simulink model "F16ASYM_Controlled"  (R2015a)
settings: Solver=ode3  SolverMode=SingleTasking  StartTime=0.0  StopTime=inf  FixedStep=T_sim  RelTol=1e-3
InitFcn:
  | load('NN_c_weights_Last_stable.mat')
StopFcn:
  | Final_results
values from neighbouring files (symbols this model uses):
  a1 = fitresult.p1    [Stall_protection.m]
  alpha_map_eval = ones(size(M_eval))*NaN    [Auto_trim_aid.m]    (also in Autotrim_maps.mat = [nan nan 0.277598136245 0.119432432992 0.0579479097061 0.027)
  beta_map_eval = ones(size(M_eval))*NaN    [Auto_trim_aid.m]    (also in Autotrim_maps.mat = [nan nan -0.00151549403324 0.00117807579006 -0.0052086799721)
  C_L_0 = fitresult.p2    [Stall_protection.m]
  G_eval = NaN*ones(size(M_sq,2),size(H_sq,2))    [Stall_protection.m]
  H_sq = unique(sort(H_sq))    [Stall_protection.m]
  H_sq_autotrim = min( F_envelope.H_1g):2000:max(F_envelope.H_1g)    [Auto_trim_aid.m]    (also in Autotrim_maps.mat = [0 2000 4000 6000 8000 10000 12000 14000 16000 18000])
  K_b_q_extrap_ACC = K_b_q_extrap    [RUN_ME.m]
  K_b_q_extrap_AoA = K_b_q_extrap    [RUN_ME.m]
  M_sq = unique(sort(M_sq))    [Stall_protection.m]
  M_sq_autotrim = 0:0.1:max(F_envelope.M_1g)    [Auto_trim_aid.m]    (also in Autotrim_maps.mat = [0 0.1 0.2 0.3 0.4 0.5 0.6 0.7 0.8 0.9 1 1.1 ... (21 element)
  T_sim = 0.02    [RUN_ME.m]
  tau_q_extrap_ACC = tau_q_extrap    [RUN_ME.m]
  tau_q_extrap_AoA = tau_q_extrap    [RUN_ME.m]
  velocity = M_eval(I,J)*a    [Auto_trim_aid.m]
undefined symbols (not defined in the file or in its folder): ACCEL, B, Earth, fi_flag_Simulink, GYRO, H_sq_sche, k_B, K_b_ACC_extrap, K_b_AoA_extrap, latitude, longitude, m, m_B, M_sq_sche, Model_used_flag, rad, s, sigbuilder_block, Stall_curve, tau_ACC_extrap, tau_AoA_extrap, Theta_1_roll_last, Theta_2_roll_last, Theta_3_roll_last, trim_control, trim_state, trim_throttle, V_Comp_A_w_z_last, V_Comp_last, V_Comp_last_ONE, V_long_lastA_w_z, V_long_lastAoA, V_roll_last, V_roll_lastMOD, V_yaw_last, W_Comp_A_w_z_last, W_Comp_last, W_long_lastA_w_z, W_long_lastAoA, W_roll_last, W_roll_lastMOD, W_yaw_last, WGS84
libraries: Adaptive_FaultTolerantControl x57, dspsigops x37, F16_Actuator_Library x14, commnoisgen2 x13, simulink x11, simulink_extras x10, dsparch4 x6, aerolibatmos2 x6, aerolibtransform2 x6, aerolibfltsims x3, dspvision x3, dspsnks4 x3
(part 5 of 14)

== system F16ASYM_Controlled/Primary Controller/P con  + Crossed NN + AWU+Lim + hand-over+Scheduling/P controller + adaptive Crossed NN + AWU+Lim    in ACC  ==
  A_w_z des : Inport
  AoA des (rad) : Inport  Port=2
  p des (rad/s) : Inport  Port=3
  beta des (rad) : Inport  Port=4
  Anti-windup A_w_z : Inport  Port=5
  Anti-windup AoA : Inport  Port=6
  Anti-windup beta : Inport  Port=7
  All measures : Inport  Port=8
  Anti-windup signals : Inport  Port=9
  Active : Inport  Port=10
  Body Rates Controller : Subsystem
  Bus Creator : BusCreator  Inputs=3
  Bus Creator1 : BusCreator  Inputs=2
  Bus Creator2 : BusCreator
  Bus Creator3 : BusCreator  Inputs=2
  Bus Selector3 : BusSelector  OutputSignals=signal1.SS meas (rad)
  Complete crossed On-line (adaptive) multi-layer NN: A_w_z : Subsystem  VariantControl=NN on A_w_z
  Display{,1..3,5..6} (6 alike) : Display
  "Display4 " : Display
  Lat_dir Dyn Inversion: beta_dot->r_c : Subsystem
  Long Dyn Inversion: alpha_dot ->q : Subsystem
  Longitudinal controller in A_w_z : Subsystem  VariantControl=Controller of A_w_z
  Memory : Memory  X0=[0,0,0]
  Physical limitation : Subsystem
  Ref Model and P Controller : Adaptive_FaultTolerantControl/Ref Model and P Controller  tau=0.45  y_i=trim_state(9)  K_f=1  K_b=5
  Scope1 : Scope
      settings: TimeRange=10  YMin=-1  YMax=1  SaveName=ScopeData27
  "Sigmoid " : Subsystem  mask{a=0.15}
      mask prompts: a "Sigmoid a param"
      mask TypeOptions a: a/Value
      mask Display:
      | x=-25:0.1:25;
      | 
      | y=(2.0 ./ (1.0 + exp(-a.*x))-1) ;
      | y2=zeros(size(x));
      | 
      | plot(x,y,x,y2);
      | 
      | text(-12,0.5, ['a= ',num2str(a)])
  Sum : Sum  Inputs=-+|
  Sum1 : Sum  Inputs=+-|
  Terminator1 : Terminator
  Angular acc des : Outport
  wires:
  Active/1 -> Complete crossed On-line (adaptive) multi-layer NN: A_w_z/Enable
  Physical limitation/1(v limted) -> Angular acc des/1
  Anti-windup signals/1 -> Complete crossed On-line (adaptive) multi-layer NN: A_w_z/4(AWU)
  Ref Model and P Controller/1 -> Lat_dir Dyn Inversion: beta_dot->r_c/1(beta_dot_c), Display5/1
  Complete crossed On-line (adaptive) multi-layer NN: A_w_z/1(v_ad^) -> Sum/1, Display2/1, Scope1/1  "v_ad^"
  "Sigmoid "/1(Out) -> Memory/1
  Anti-windup beta/1 -> Terminator1/1
  Bus Creator3/1 -> Bus Creator/3  "beta_r_chanel"
  Bus Creator2/1 -> Bus Creator3/2  "beta_chanel vars"
  Body Rates Controller/3(r_chanel vars) -> Bus Creator3/1  "r_chanel vars"
  Ref Model and P Controller/5 -> Bus Creator2/4  "K_b_beta"
  Ref Model and P Controller/4 -> Sum1/2
  Sum1/1 -> Bus Creator2/3  "beta_err"
  Ref Model and P Controller/3 -> Bus Creator2/2, Sum1/1  "beta_sf"
  Ref Model and P Controller/2 -> Bus Creator2/1  "beta_sf_dot"
  Bus Creator1/1 -> Bus Creator/1  "Long chanel"
  Longitudinal controller in A_w_z/1(A_chanel vars) -> Bus Creator1/1  "A_chanel vars"
  Body Rates Controller/1(q_chanel vars) -> Bus Creator1/2  "q_chanel_vars"
  Body Rates Controller/2(p_chanel vars) -> Bus Creator/2  "p_chanel_vars"
  Memory/1 -> Complete crossed On-line (adaptive) multi-layer NN: A_w_z/1(v_ad^ prev)
  Bus Creator/1 -> Complete crossed On-line (adaptive) multi-layer NN: A_w_z/3(NN variables)
  Body Rates Controller/4(Angular acc des (rad/s^2)) -> Sum/2, Display3/1  "v_p+v_dot_ff"
  All measures/1 -> Longitudinal controller in A_w_z/5(All meas), Long Dyn Inversion: alpha_dot ->q/2(All_meas), Bus Selector3/1, Lat_dir Dyn Inversion: beta_dot->r_c/2(All_meas), Body Rates Controller/4(All_meas), Physical limitation/2(all meas), Complete crossed On-line (adaptive) multi-layer NN: A_w_z/2(All_meas)
  Sum/1 -> Physical limitation/1(v comm), "Sigmoid "/1(In), "Display4 "/1  "v"
  A_w_z des/1 -> Longitudinal controller in A_w_z/1(A_w_z des)
  Anti-windup A_w_z/1 -> Longitudinal controller in A_w_z/3(Anti-windup A_w_z)
  Anti-windup AoA/1 -> Longitudinal controller in A_w_z/4(Anti-windup AoA)
  AoA des (rad)/1 -> Longitudinal controller in A_w_z/2(AoA des (rad))
  Longitudinal controller in A_w_z/2(alpha_dot_c) -> Display/1, Long Dyn Inversion: alpha_dot ->q/1(alpha_dot_c)
  beta des (rad)/1 -> Ref Model and P Controller/1
  Long Dyn Inversion: alpha_dot ->q/1(q_c) -> Display1/1, Body Rates Controller/2(q_ref)
  p des (rad/s)/1 -> Body Rates Controller/1(p_ref)
  Bus Selector3/1 -> Ref Model and P Controller/2  "<SS meas (rad)>"
  Lat_dir Dyn Inversion: beta_dot->r_c/1(r_c) -> Body Rates Controller/3(r_ref), Display6/1

== system F16ASYM_Controlled/Primary Controller/P con  + Crossed NN + AWU+Lim + hand-over+Scheduling/P controller + adaptive Crossed NN + AWU+Lim   in AoA ==
  A_w_z des : Inport
  AoA des (rad) : Inport  Port=2
  p des (rad/s) : Inport  Port=3
  beta des (rad) : Inport  Port=4
  Anti-windup A_w_z : Inport  Port=5
  Anti-windup AoA : Inport  Port=6
  Anti-windup beta : Inport  Port=7
  All measures : Inport  Port=8
  Anti-windup signals : Inport  Port=9
  Active : Inport  Port=10
  Body Rates Controller : Subsystem
  Bus Creator : BusCreator  Inputs=3
  Bus Creator1 : BusCreator  Inputs=2
  Bus Creator2 : BusCreator
  Bus Creator3 : BusCreator  Inputs=2
  Bus Selector3 : BusSelector  OutputSignals=signal1.SS meas (rad)
  Complete crossed On-line (adaptive) multi-layer NN: AoA : Subsystem  VariantControl=NN on AoA
  Display{,1..3,5..6} (6 alike) : Display
  "Display4 " : Display
  Lat_dir Dyn Inversion: beta_dot->r_c : Subsystem
  Long Dyn Inversion: alpha_dot ->q : Subsystem
  Longitudinal controller in AoA1 : Subsystem  VariantControl=Controller of AoA
  Memory : Memory  X0=[0,0,0]
  Physical limitation : Subsystem
  Ref Model and P Controller : Adaptive_FaultTolerantControl/Ref Model and P Controller  tau=0.45  y_i=trim_state(9)  K_f=1  K_b=5
  Scope1 : Scope
      settings: YMin=-8000  YMax=9000  SaveName=ScopeData27
  "Sigmoid " : Subsystem  mask{a=0.15}
      mask prompts: a "Sigmoid a param"
      mask TypeOptions a: a/Value
      mask Display:
      | x=-25:0.1:25;
      | 
      | y=(2.0 ./ (1.0 + exp(-a.*x))-1) ;
      | y2=zeros(size(x));
      | 
      | plot(x,y,x,y2);
      | 
      | text(-12,0.5, ['a= ',num2str(a)])
  Sum : Sum  Inputs=-+|
  Sum1 : Sum  Inputs=+-|
  Terminator1 : Terminator
  Angular acc des : Outport
  wires:
  Active/1 -> Complete crossed On-line (adaptive) multi-layer NN: AoA/Enable
  Anti-windup signals/1 -> Complete crossed On-line (adaptive) multi-layer NN: AoA/4(AWU)
  Physical limitation/1(v limted) -> Angular acc des/1
  Ref Model and P Controller/1 -> Lat_dir Dyn Inversion: beta_dot->r_c/1(beta_dot_c), Display5/1
  Complete crossed On-line (adaptive) multi-layer NN: AoA/1(v_ad^) -> Sum/1, Display2/1, Scope1/1  "v_ad^"
  "Sigmoid "/1(Out) -> Memory/1
  Anti-windup beta/1 -> Terminator1/1
  Bus Creator3/1 -> Bus Creator/3  "beta_r_chanel"
  Bus Creator2/1 -> Bus Creator3/2  "beta_chanel vars"
  Body Rates Controller/3(r_chanel vars) -> Bus Creator3/1  "r_chanel vars"
  Ref Model and P Controller/5 -> Bus Creator2/4  "K_b_beta"
  Ref Model and P Controller/4 -> Sum1/2
  Sum1/1 -> Bus Creator2/3  "beta_err"
  Ref Model and P Controller/3 -> Bus Creator2/2, Sum1/1  "beta_sf"
  Ref Model and P Controller/2 -> Bus Creator2/1  "beta_sf_dot"
  Bus Creator1/1 -> Bus Creator/1  "Long chanel"
  Longitudinal controller in AoA1/1(alpha_chanel vars) -> Bus Creator1/1  "alpha_chanel vars"
  Body Rates Controller/1(q_chanel vars) -> Bus Creator1/2  "q_chanel_vars"
  Body Rates Controller/2(p_chanel vars) -> Bus Creator/2  "p_chanel_vars"
  Memory/1 -> Complete crossed On-line (adaptive) multi-layer NN: AoA/1(v_ad^ prev)
  Bus Creator/1 -> Complete crossed On-line (adaptive) multi-layer NN: AoA/3(NN variables)
  Body Rates Controller/4(Angular acc des (rad/s^2)) -> Sum/2, Display3/1  "v_p+v_dot_ff"
  All measures/1 -> Longitudinal controller in AoA1/5(All meas), Long Dyn Inversion: alpha_dot ->q/2(All_meas), Bus Selector3/1, Lat_dir Dyn Inversion: beta_dot->r_c/2(All_meas), Body Rates Controller/4(All_meas), Physical limitation/2(all meas), Complete crossed On-line (adaptive) multi-layer NN: AoA/2(All_meas)
  Sum/1 -> Physical limitation/1(v comm), "Sigmoid "/1(In), "Display4 "/1  "v"
  A_w_z des/1 -> Longitudinal controller in AoA1/1(A_w_z des)
  Anti-windup A_w_z/1 -> Longitudinal controller in AoA1/3(Anti-windup A_w_z)
  Anti-windup AoA/1 -> Longitudinal controller in AoA1/4(Anti-windup AoA)
  AoA des (rad)/1 -> Longitudinal controller in AoA1/2(AoA des (rad))
  Longitudinal controller in AoA1/2(alpha_dot_c) -> Display/1, Long Dyn Inversion: alpha_dot ->q/1(alpha_dot_c)
  beta des (rad)/1 -> Ref Model and P Controller/1
  Long Dyn Inversion: alpha_dot ->q/1(q_c) -> Display1/1, Body Rates Controller/2(q_ref)
  p des (rad/s)/1 -> Body Rates Controller/1(p_ref)
  Bus Selector3/1 -> Ref Model and P Controller/2  "<SS meas (rad)>"
  Lat_dir Dyn Inversion: beta_dot->r_c/1(r_c) -> Body Rates Controller/3(r_ref), Display6/1

== system F16ASYM_Controlled/Primary Controller/P con  + Crossed NN + AWU+Lim + hand-over+Scheduling/Transitions Smoother  ==
  note: When changing here the time, be careful and change also
      | the denominator of the gains of the inputs of the integrators
  From AoA : Inport
  Indicator : Inport  Port=2
  From  ACC : Inport  Port=3
  "ACC -> AoA" : Saturate  UpperLimit=1  LowerLimit=0
  Abs : Abs
  Abs1 : Abs
  Add : Sum  Inputs=+-  OutDataTypeStr=double
  Add1 : Sum  Inputs=+-
  Add2 : Sum  Inputs=-+
  Add3 : Sum  Inputs=-+
  Add4 : Sum  Inputs=+-
  Add6 : Sum  Inputs=+-
  Add7 : Sum  Commented=on  Inputs=+-
  "AoA -> ACC" : Saturate  UpperLimit=0  LowerLimit=-1
  Divide : Product  Inputs=**
  Divide1 : Product  Inputs=**
  Gain1 : Gain  Gain=-1/1
  Gain2 : Gain  Gain=-1/1
  Integrator Limited1 : Integrator  ExternalReset=level  InitialConditionSource=external  LimitOutput=on  UpperSaturationLimit=100  LowerSaturationLimit=-100
  Integrator Limited2 : Integrator  ExternalReset=level  InitialConditionSource=external  LimitOutput=on  UpperSaturationLimit=100  LowerSaturationLimit=-100
  Logical Operator : Logic  Operator=NOT  IconShape=distinctive  AllPortsSameDT=off  OutDataTypeStr=boolean
  Logical Operator1 : Logic  Operator=NOT  IconShape=distinctive  AllPortsSameDT=off  OutDataTypeStr=boolean
  Logical Operator2 : Logic  Operator=NOT  IconShape=distinctive  AllPortsSameDT=off  OutDataTypeStr=boolean
  Sample and Hold{1..4} (4 alike) : dspsigops/Sample and Hold  trig=Either edge  initCond=0  latchinput=off
  Scope3 : Scope
      settings: SaveName=ScopeData36
  Scope4 : Scope
      settings: YMin=-0.08  YMax=0.02  SaveName=ScopeData37
  Switch : Switch  Threshold=0.5  InputSameDT=on
  Timer signal : Subsystem  mask{time_delay=1}
      mask prompts: time_delay "Time to delay (s)"
  Unit Delay : UnitDelay  SampleTime=-1
  Ang accels comm : Outport
  wires:
  Logical Operator2/1 -> Divide1/1
  Divide1/1 -> Add6/2, Scope3/1
  Divide/1 -> Scope4/1, Add4/2
  Logical Operator1/1 -> Divide/1
  Gain2/1 -> Integrator Limited2/1
  Gain1/1 -> Integrator Limited1/1
  Sample and Hold4/1 -> Add7/2
  "ACC -> AoA"/1 -> Sample and Hold4/Trigger, Sample and Hold3/Trigger
  Integrator Limited2/1 -> Divide1/2
  Add6/1 -> Switch/1
  Switch/1 -> Ang accels comm/1
  Logical Operator/1 -> Logical Operator1/1, Integrator Limited1/2, Logical Operator2/1, Integrator Limited2/2
  Add4/1 -> Switch/3
  Integrator Limited1/1 -> Divide/2
  Sample and Hold2/1 -> Add3/1
  Add3/1 -> Gain1/1
  Sample and Hold1/1 -> Integrator Limited1/3
  Add2/1 -> Sample and Hold1/1
  Abs/1 -> Sample and Hold2/Trigger, Sample and Hold1/Trigger
  From AoA/1 -> Add1/1, Add6/1, Add7/1, Add2/1, Sample and Hold2/1
  Add1/1 -> Sample and Hold3/1
  "AoA -> ACC"/1 -> Abs/1
  Add/1 -> Abs1/1, "ACC -> AoA"/1, "AoA -> ACC"/1
  From  ACC/1 -> Add1/2, Sample and Hold4/1, Add4/1, Add2/2, Add3/2
  Timer signal/1(Logic output) -> Logical Operator/1
  Abs1/1 -> Timer signal/1(Triger)
  Unit Delay/1 -> Add/2
  Indicator/1 -> Add/1, Unit Delay/1, Switch/2
  Sample and Hold3/1 -> Gain2/1, Integrator Limited2/3

== system F16ASYM_Controlled/Primary Controller/P con + Crossed NN + AWU+Lim + hand-over/P controller + adaptive Crossed NN + AWU+Lim    in ACC  ==
  A_w_z des : Inport
  AoA des (rad) : Inport  Port=2
  p des (rad/s) : Inport  Port=3
  beta des (rad) : Inport  Port=4
  Anti-windup A_w_z : Inport  Port=5
  Anti-windup AoA : Inport  Port=6
  Anti-windup beta : Inport  Port=7
  All measures : Inport  Port=8
  Anti-windup signals : Inport  Port=9
  Active : Inport  Port=10
  Body Rates Controller : Subsystem
  Bus Creator : BusCreator  Inputs=3
  Bus Creator1 : BusCreator  Inputs=2
  Bus Creator2 : BusCreator
  Bus Creator3 : BusCreator  Inputs=2
  Bus Selector3 : BusSelector  OutputSignals=signal1.SS meas (rad)
  Complete crossed On-line (adaptive) multi-layer NN: A_w_z : Subsystem  VariantControl=NN on A_w_z
  Display{,1..3,5..6} (6 alike) : Display
  "Display4 " : Display
  Lat_dir Dyn Inversion: beta_dot->r_c : Subsystem
  Long Dyn Inversion: alpha_dot ->q : Subsystem
  Longitudinal controller in A_w_z : Subsystem  VariantControl=Controller of A_w_z
  Memory : Memory  X0=[0,0,0]
  Physical limitation : Subsystem
  Ref Model and P Controller : Adaptive_FaultTolerantControl/Ref Model and P Controller  tau=0.45  y_i=trim_state(9)  K_f=1  K_b=5
  Scope1 : Scope
      settings: TimeRange=10  YMin=-1  YMax=1  SaveName=ScopeData27
  "Sigmoid " : Subsystem  mask{a=0.15}
      mask prompts: a "Sigmoid a param"
      mask TypeOptions a: a/Value
      mask Display:
      | x=-25:0.1:25;
      | 
      | y=(2.0 ./ (1.0 + exp(-a.*x))-1) ;
      | y2=zeros(size(x));
      | 
      | plot(x,y,x,y2);
      | 
      | text(-12,0.5, ['a= ',num2str(a)])
  Sum : Sum  Inputs=-+|
  Sum1 : Sum  Inputs=+-|
  Terminator1 : Terminator
  Angular acc des : Outport
  wires:
  Lat_dir Dyn Inversion: beta_dot->r_c/1(r_c) -> Display6/1, Body Rates Controller/3(r_ref)
  Bus Selector3/1 -> Ref Model and P Controller/2  "<SS meas (rad)>"
  p des (rad/s)/1 -> Body Rates Controller/1(p_ref)
  Long Dyn Inversion: alpha_dot ->q/1(q_c) -> Body Rates Controller/2(q_ref), Display1/1
  beta des (rad)/1 -> Ref Model and P Controller/1
  Longitudinal controller in A_w_z/2(alpha_dot_c) -> Long Dyn Inversion: alpha_dot ->q/1(alpha_dot_c), Display/1
  AoA des (rad)/1 -> Longitudinal controller in A_w_z/2(AoA des (rad))
  Anti-windup AoA/1 -> Longitudinal controller in A_w_z/4(Anti-windup AoA)
  Anti-windup A_w_z/1 -> Longitudinal controller in A_w_z/3(Anti-windup A_w_z)
  A_w_z des/1 -> Longitudinal controller in A_w_z/1(A_w_z des)
  Sum/1 -> "Display4 "/1, "Sigmoid "/1(In), Physical limitation/1(v comm)  "v"
  All measures/1 -> Complete crossed On-line (adaptive) multi-layer NN: A_w_z/2(All_meas), Physical limitation/2(all meas), Body Rates Controller/4(All_meas), Lat_dir Dyn Inversion: beta_dot->r_c/2(All_meas), Bus Selector3/1, Long Dyn Inversion: alpha_dot ->q/2(All_meas), Longitudinal controller in A_w_z/5(All meas)
  Body Rates Controller/4(Angular acc des (rad/s^2)) -> Display3/1, Sum/2  "v_p+v_dot_ff"
  Bus Creator/1 -> Complete crossed On-line (adaptive) multi-layer NN: A_w_z/3(NN variables)
  Memory/1 -> Complete crossed On-line (adaptive) multi-layer NN: A_w_z/1(v_ad^ prev)
  Body Rates Controller/2(p_chanel vars) -> Bus Creator/2  "p_chanel_vars"
  Body Rates Controller/1(q_chanel vars) -> Bus Creator1/2  "q_chanel_vars"
  Longitudinal controller in A_w_z/1(A_chanel vars) -> Bus Creator1/1  "A_chanel vars"
  Bus Creator1/1 -> Bus Creator/1  "Long chanel"
  Ref Model and P Controller/2 -> Bus Creator2/1  "beta_sf_dot"
  Ref Model and P Controller/3 -> Sum1/1, Bus Creator2/2  "beta_sf"
  Sum1/1 -> Bus Creator2/3  "beta_err"
  Ref Model and P Controller/4 -> Sum1/2
  Ref Model and P Controller/5 -> Bus Creator2/4  "K_b_beta"
  Body Rates Controller/3(r_chanel vars) -> Bus Creator3/1  "r_chanel vars"
  Bus Creator2/1 -> Bus Creator3/2  "beta_chanel vars"
  Bus Creator3/1 -> Bus Creator/3  "beta_r_chanel"
  Anti-windup beta/1 -> Terminator1/1
  "Sigmoid "/1(Out) -> Memory/1
  Complete crossed On-line (adaptive) multi-layer NN: A_w_z/1(v_ad^) -> Scope1/1, Display2/1, Sum/1  "v_ad^"
  Ref Model and P Controller/1 -> Display5/1, Lat_dir Dyn Inversion: beta_dot->r_c/1(beta_dot_c)
  Anti-windup signals/1 -> Complete crossed On-line (adaptive) multi-layer NN: A_w_z/4(AWU)
  Physical limitation/1(v limted) -> Angular acc des/1
  Active/1 -> Complete crossed On-line (adaptive) multi-layer NN: A_w_z/Enable

== system F16ASYM_Controlled/Primary Controller/P con + Crossed NN + AWU+Lim + hand-over/P controller + adaptive Crossed NN + AWU+Lim   in AoA ==
  A_w_z des : Inport
  AoA des (rad) : Inport  Port=2
  p des (rad/s) : Inport  Port=3
  beta des (rad) : Inport  Port=4
  Anti-windup A_w_z : Inport  Port=5
  Anti-windup AoA : Inport  Port=6
  Anti-windup beta : Inport  Port=7
  All measures : Inport  Port=8
  Anti-windup signals : Inport  Port=9
  Active : Inport  Port=10
  Body Rates Controller : Subsystem
  Bus Creator : BusCreator  Inputs=3
  Bus Creator1 : BusCreator  Inputs=2
  Bus Creator2 : BusCreator
  Bus Creator3 : BusCreator  Inputs=2
  Bus Selector3 : BusSelector  OutputSignals=signal1.SS meas (rad)
  Complete crossed On-line (adaptive) multi-layer NN: AoA : Subsystem  VariantControl=NN on AoA
  Display{,1..3,5..6} (6 alike) : Display
  "Display4 " : Display
  Lat_dir Dyn Inversion: beta_dot->r_c : Subsystem
  Long Dyn Inversion: alpha_dot ->q : Subsystem
  Longitudinal controller in AoA : Subsystem  VariantControl=Controller of AoA
  Memory : Memory  X0=[0,0,0]
  Physical limitation : Subsystem
  Ref Model and P Controller : Adaptive_FaultTolerantControl/Ref Model and P Controller  tau=0.45  y_i=trim_state(9)  K_f=1  K_b=5
  Scope1 : Scope
      settings: YMin=-8000  YMax=9000  SaveName=ScopeData27
  "Sigmoid " : Subsystem  mask{a=0.15}
      mask prompts: a "Sigmoid a param"
      mask TypeOptions a: a/Value
      mask Display:
      | x=-25:0.1:25;
      | 
      | y=(2.0 ./ (1.0 + exp(-a.*x))-1) ;
      | y2=zeros(size(x));
      | 
      | plot(x,y,x,y2);
      | 
      | text(-12,0.5, ['a= ',num2str(a)])
  Sum : Sum  Inputs=-+|
  Sum1 : Sum  Inputs=+-|
  Terminator1 : Terminator
  Angular acc des : Outport
  wires:
  Lat_dir Dyn Inversion: beta_dot->r_c/1(r_c) -> Display6/1, Body Rates Controller/3(r_ref)
  Bus Selector3/1 -> Ref Model and P Controller/2  "<SS meas (rad)>"
  p des (rad/s)/1 -> Body Rates Controller/1(p_ref)
  Long Dyn Inversion: alpha_dot ->q/1(q_c) -> Body Rates Controller/2(q_ref), Display1/1
  beta des (rad)/1 -> Ref Model and P Controller/1
  Longitudinal controller in AoA/2(alpha_dot_c) -> Long Dyn Inversion: alpha_dot ->q/1(alpha_dot_c), Display/1
  AoA des (rad)/1 -> Longitudinal controller in AoA/2(AoA des (rad))
  Anti-windup AoA/1 -> Longitudinal controller in AoA/4(Anti-windup AoA)
  Anti-windup A_w_z/1 -> Longitudinal controller in AoA/3(Anti-windup A_w_z)
  A_w_z des/1 -> Longitudinal controller in AoA/1(A_w_z des)
  Sum/1 -> "Display4 "/1, "Sigmoid "/1(In), Physical limitation/1(v comm)  "v"
  All measures/1 -> Complete crossed On-line (adaptive) multi-layer NN: AoA/2(All_meas), Longitudinal controller in AoA/5(All meas), Physical limitation/2(all meas), Body Rates Controller/4(All_meas), Lat_dir Dyn Inversion: beta_dot->r_c/2(All_meas), Bus Selector3/1, Long Dyn Inversion: alpha_dot ->q/2(All_meas)
  Body Rates Controller/4(Angular acc des (rad/s^2)) -> Display3/1, Sum/2  "v_p+v_dot_ff"
  Bus Creator/1 -> Complete crossed On-line (adaptive) multi-layer NN: AoA/3(NN variables)
  Memory/1 -> Complete crossed On-line (adaptive) multi-layer NN: AoA/1(v_ad^ prev)
  Body Rates Controller/2(p_chanel vars) -> Bus Creator/2  "p_chanel_vars"
  Body Rates Controller/1(q_chanel vars) -> Bus Creator1/2  "q_chanel_vars"
  Longitudinal controller in AoA/1(alpha_chanel vars) -> Bus Creator1/1  "alpha_chanel vars"
  Bus Creator1/1 -> Bus Creator/1  "Long chanel"
  Ref Model and P Controller/2 -> Bus Creator2/1  "beta_sf_dot"
  Ref Model and P Controller/3 -> Sum1/1, Bus Creator2/2  "beta_sf"
  Sum1/1 -> Bus Creator2/3  "beta_err"
  Ref Model and P Controller/4 -> Sum1/2
  Ref Model and P Controller/5 -> Bus Creator2/4  "K_b_beta"
  Body Rates Controller/3(r_chanel vars) -> Bus Creator3/1  "r_chanel vars"
  Bus Creator2/1 -> Bus Creator3/2  "beta_chanel vars"
  Bus Creator3/1 -> Bus Creator/3  "beta_r_chanel"
  Anti-windup beta/1 -> Terminator1/1
  "Sigmoid "/1(Out) -> Memory/1
  Complete crossed On-line (adaptive) multi-layer NN: AoA/1(v_ad^) -> Scope1/1, Display2/1, Sum/1  "v_ad^"
  Ref Model and P Controller/1 -> Display5/1, Lat_dir Dyn Inversion: beta_dot->r_c/1(beta_dot_c)
  Physical limitation/1(v limted) -> Angular acc des/1
  Anti-windup signals/1 -> Complete crossed On-line (adaptive) multi-layer NN: AoA/4(AWU)
  Active/1 -> Complete crossed On-line (adaptive) multi-layer NN: AoA/Enable

== system F16ASYM_Controlled/Primary Controller/P con + Crossed NN + AWU+Lim + hand-over/Transitions Smoother  ==
  note: When changing here the time, be careful and change also
      | the denominator of the gains of the inputs of the integrators
  From AoA : Inport
  Indicator : Inport  Port=2
  From  ACC : Inport  Port=3
  "ACC -> AoA" : Saturate  UpperLimit=1  LowerLimit=0
  Abs : Abs
  Abs1 : Abs
  Add : Sum  Inputs=+-  OutDataTypeStr=double
  Add{1,4,6..7} (4 alike) : Sum  Inputs=+-
  Add2 : Sum  Inputs=-+
  Add3 : Sum  Inputs=-+
  "AoA -> ACC" : Saturate  UpperLimit=0  LowerLimit=-1
  Divide : Product  Inputs=**
  Divide1 : Product  Inputs=**
  Gain1 : Gain  Gain=-1/1
  Gain2 : Gain  Gain=-1/1
  Integrator Limited1 : Integrator  ExternalReset=level  InitialConditionSource=external  LimitOutput=on  UpperSaturationLimit=100  LowerSaturationLimit=-100
  Integrator Limited2 : Integrator  ExternalReset=level  InitialConditionSource=external  LimitOutput=on  UpperSaturationLimit=100  LowerSaturationLimit=-100
  Logical Operator : Logic  Operator=NOT  IconShape=distinctive  AllPortsSameDT=off  OutDataTypeStr=boolean
  Logical Operator1 : Logic  Operator=NOT  IconShape=distinctive  AllPortsSameDT=off  OutDataTypeStr=boolean
  Logical Operator2 : Logic  Operator=NOT  IconShape=distinctive  AllPortsSameDT=off  OutDataTypeStr=boolean
  Sample and Hold{1..4} (4 alike) : dspsigops/Sample and Hold  trig=Either edge  initCond=0  latchinput=off
  Scope{1..4} (4 alike) : Scope
      Scope1 settings: SaveName=ScopeData35
      Scope2 settings: SaveName=ScopeData34
      Scope3 settings: SaveName=ScopeData36
      Scope4 settings: YMin=-0.08  YMax=0.02  SaveName=ScopeData37
  Switch : Switch  Threshold=0.5  InputSameDT=on
  Timer signal : Subsystem  mask{time_delay=1}
      mask prompts: time_delay "Time to delay (s)"
  Unit Delay : UnitDelay  SampleTime=-1
  Ang accels comm : Outport
  wires:
  Indicator/1 -> Switch/2, Unit Delay/1, Add/1
  Unit Delay/1 -> Add/2
  Abs1/1 -> Timer signal/1(Triger)
  Timer signal/1(Logic output) -> Logical Operator/1
  From  ACC/1 -> Add3/2, Add2/2, Add4/1, Sample and Hold4/1, Add1/2
  Add/1 -> "AoA -> ACC"/1, "ACC -> AoA"/1, Abs1/1
  "AoA -> ACC"/1 -> Abs/1
  Add1/1 -> Sample and Hold3/1
  From AoA/1 -> Sample and Hold2/1, Add2/1, Add7/1, Add6/1, Add1/1
  Abs/1 -> Sample and Hold1/Trigger, Sample and Hold2/Trigger
  Add2/1 -> Sample and Hold1/1
  Sample and Hold1/1 -> Integrator Limited1/3
  Add3/1 -> Gain1/1
  Sample and Hold2/1 -> Add3/1
  Integrator Limited1/1 -> Divide/2
  Add4/1 -> Switch/3
  Logical Operator/1 -> Integrator Limited2/2, Logical Operator2/1, Integrator Limited1/2, Logical Operator1/1, Scope2/1
  Switch/1 -> Scope1/1, Ang accels comm/1
  Add6/1 -> Switch/1
  Integrator Limited2/1 -> Divide1/2
  "ACC -> AoA"/1 -> Sample and Hold3/Trigger, Sample and Hold4/Trigger
  Sample and Hold4/1 -> Add7/2
  Gain1/1 -> Integrator Limited1/1
  Gain2/1 -> Integrator Limited2/1
  Logical Operator1/1 -> Divide/1
  Divide/1 -> Add4/2, Scope4/1
  Divide1/1 -> Scope3/1, Add6/2
  Logical Operator2/1 -> Divide1/1
  Sample and Hold3/1 -> Gain2/1, Integrator Limited2/3

== system F16ASYM_Controlled/Primary Controller/P con + Crossed NN + AWU+Lim + hand-over/Transitions Smotother 1 ==
  From AoA : Inport
  Indicator : Inport  Port=2
  From  ACC : Inport  Port=3
  "ACC -> AoA" : Saturate  UpperLimit=1  LowerLimit=0
  Abs : Abs
  Add : Sum  Inputs=+-  OutDataTypeStr=double
  Add1 : Sum  Inputs=+-
  Add2 : Sum  Inputs=-+
  Add3 : Sum  Inputs=+-
  Add5 : Sum  Inputs=+-
  "AoA -> ACC" : Saturate  UpperLimit=0  LowerLimit=-1
  Gain : Gain  Gain=-1/5
  Gain1 : Gain  Gain=-1/5
  Integrator Limited : Integrator  ExternalReset=rising  InitialConditionSource=external  LimitOutput=on  UpperSaturationLimit=10000  LowerSaturationLimit=0
  Integrator Limited1 : Integrator  ExternalReset=rising  InitialConditionSource=external  LimitOutput=on  UpperSaturationLimit=100  LowerSaturationLimit=0
  Sample and Hold1 : dspsigops/Sample and Hold  trig=Rising edge  initCond=0  latchinput=off
  Sample and Hold2 : dspsigops/Sample and Hold  trig=Rising edge  initCond=0  latchinput=off
  Scope4 : Scope
      settings: YMin=-4  YMax=1.5  SaveName=ScopeData38
  Switch : Switch  Threshold=0.5  InputSameDT=on
  Unit Delay : UnitDelay  SampleTime=-1
  Out1 : Outport
  wires:
  Switch/1 -> Out1/1
  Gain1/1 -> Integrator Limited1/1
  Gain/1 -> Integrator Limited/1
  Add5/1 -> Switch/3
  Sample and Hold1/1 -> Integrator Limited1/3, Gain1/1
  Abs/1 -> Integrator Limited1/2, Sample and Hold1/Trigger
  Integrator Limited1/1 -> Add5/2
  Add2/1 -> Sample and Hold1/1
  Add3/1 -> Switch/1
  Sample and Hold2/1 -> Integrator Limited/3, Gain/1
  "ACC -> AoA"/1 -> Integrator Limited/2, Sample and Hold2/Trigger
  Integrator Limited/1 -> Add3/2
  Add1/1 -> Sample and Hold2/1
  "AoA -> ACC"/1 -> Abs/1
  Add/1 -> "AoA -> ACC"/1, "ACC -> AoA"/1
  From  ACC/1 -> Add1/2, Add5/1, Add2/2
  From AoA/1 -> Add2/1, Add1/1, Add3/1, Scope4/1
  Unit Delay/1 -> Add/2
  Indicator/1 -> Add/1, Unit Delay/1, Switch/2

== system F16ASYM_Controlled/Primary Controller/P con + adaptive Crossed NN + AWU+Lim + Scheduling/Body Rates Controller ==
  p_ref : Inport
  q_ref : Inport  Port=2
  r_ref : Inport  Port=3
  All_meas : Inport  Port=4
  Body Rates Controller  in ACC : Subsystem  VariantControl=Body rates controller of ACC
  Body Rates Controller in  AoA : Subsystem  VariantControl=Body rates controller of AoA
  q_chanel vars : Outport
  p_chanel vars : Outport  Port=2
  r_chanel vars : Outport  Port=3
  Angular acc des (rad/s^2) : Outport  Port=4

== system F16ASYM_Controlled/Primary Controller/P con + adaptive Crossed NN + AWU+Lim + Scheduling/Complete crossed On-line (adaptive) multi-layer NN ==
  v_ad^ prev : Inport
  All_meas : Inport  Port=2
  NN variables : Inport  Port=3
  AWU : Inport  Port=4
  Complete crossed On-line (adaptive) multi-layer NN: A_w_z : Subsystem  VariantControl=NN on A_w_z
  Complete crossed On-line (adaptive) multi-layer NN: AoA : Subsystem  VariantControl=NN on AoA
  v_ad^ : Outport

== system F16ASYM_Controlled/Primary Controller/P con + adaptive Crossed NN + AWU+Lim + Scheduling/Lat_dir Dyn Inversion: beta_dot->r_c ==
  beta_dot_c : Inport
  All_meas : Inport  Port=2
  A_w_y : Selector  InputPortWidth=3  Indices=2
  Bus Selector : BusSelector  OutputSignals=signal1.AoA meas (rad),signal1.omega_b meas (rad/s),signal1.V_TAS (m/s),signal2.A_w_CG
  Divide1 : Product  Inputs=**
  Divide3 : Product  Inputs=**
  Divide4 : Product  Inputs=/*
  Divide5 : Product  Inputs=*/
  Selector : Selector  InputPortWidth=3
  Trigonometric Function : Trigonometry  Operator=cos
  Trigonometric Function3 : Trigonometry  Operator=tan
  "q_c " : Sum  Inputs=-++
  r_c : Outport
  wires:
  Selector/1 -> Divide1/2
  Trigonometric Function3/1 -> Divide1/1
  beta_dot_c/1 -> Divide5/1
  Divide5/1 -> "q_c "/1
  Trigonometric Function/1 -> Divide5/2, Divide3/1
  Bus Selector/3 -> Divide3/2  "<V_TAS (m/s)>"
  Divide4/1 -> "q_c "/3
  Bus Selector/4 -> A_w_y/1  "<A_w_CG>"
  All_meas/1 -> Bus Selector/1
  A_w_y/1 -> Divide4/2
  Divide3/1 -> Divide4/1
  Divide1/1 -> "q_c "/2
  Bus Selector/2 -> Selector/1  "<omega_b meas (rad/s)>"
  Bus Selector/1 -> Trigonometric Function3/1, Trigonometric Function/1  "<AoA meas (rad)>"
  "q_c "/1 -> r_c/1

== system F16ASYM_Controlled/Primary Controller/P con + adaptive Crossed NN + AWU+Lim + Scheduling/Long Dyn Inversion: alpha_dot ->q ==
  alpha_dot_c : Inport
  All_meas : Inport  Port=2
  Completed : Subsystem
  Manual Switch : ManualSwitch
  Simplified : Subsystem
  q_c : Outport
  wires:
  Manual Switch/1 -> q_c/1
  Simplified/1(q_c) -> Manual Switch/2
  Completed/1(q_c) -> Manual Switch/1
  All_meas/1 -> Completed/2(All_meas), Simplified/2(All_meas)
  alpha_dot_c/1 -> Completed/1(alpha_dot_c), Simplified/1(alpha_dot_c)

== system F16ASYM_Controlled/Primary Controller/P con + adaptive Crossed NN + AWU+Lim + Scheduling/Longitudinal Controller: AoA or A_w_z ==
  A_w_z des : Inport
  AoA des (rad) : Inport  Port=2
  Anti-windup A_w_z : Inport  Port=3
  Anti-windup AoA : Inport  Port=4
  All meas : Inport  Port=5
  Longitudinal controller in A_w_z : Subsystem  VariantControl=Controller of A_w_z
  Longitudinal controller in AoA : Subsystem  VariantControl=Controller of AoA
  A_chanel vars : Outport
  alpha_chanel vars : Outport  Port=2
  alpha_dot_c : Outport  Port=3

== system F16ASYM_Controlled/Primary Controller/P con + adaptive Crossed NN + AWU+Lim + Scheduling/Physical limitation ==
  note: Converto to Angular accelerations
  v comm : Inport
  all meas : Inport  Port=2
  Ang Accel : MATLAB Function
  Bus Selector : BusSelector  OutputSignals=signal1.Alt meas (m),signal1.V_TAS (m/s),signal1.AoA meas (rad),signal1.SS meas (rad),signal1.omega_b meas (rad/s),signal1.Throttle_meas
  Bus Selector1 : BusSelector  OutputSignals=signal2.q (Pa),signal1.omega_b meas (rad/s)
  Demux : Demux  Outputs=3
  Display : Display
  Display1 : Display
  Display2 : Display
  Divide : Product  Inputs=**
  Divide1 : Product  Inputs=**
  Gain : Gain  Gain=-1
  Gain1 : Gain
  Mom coefficients that was reached : MATLABFcn  MATLABFcn=Moms_Coeff_estimator  OutputDimensions=3  OutputSignalType=real
  Moments : Subsystem
  Mux : Mux  Inputs=3
  Mux1 : Mux  Inputs=7
  Saturation Dynamic : simulink/Discontinuities/Saturation Dynamic  OutMin=[]  OutMax=[]  OutDataTypeStr=Inherit: Same as second input  OutDataType=fixdt(1, 16)  OutScaling=2^-10  DoSatur=off
  Sign : Signum
  Sign1 : Signum
  max deflections estimator : MATLAB Function  TreatAsAtomicUnit=on
  v limted : Outport
  wires:
  Divide1/1 -> Saturation Dynamic/3
  Gain/1 -> Divide1/2
  Divide/1 -> Saturation Dynamic/1
  Sign1/1 -> Gain/1
  Gain1/1 -> Sign/1, Display2/1, Sign1/1, Divide1/1, Divide/2
  Sign/1 -> Divide/1
  Saturation Dynamic/1 -> v limted/1, Display/1
  v comm/1 -> max deflections estimator/1(v_comm), Display1/1, Saturation Dynamic/2
  Mux/1 -> Gain1/1
  all meas/1 -> Bus Selector1/1, Bus Selector/1
  Mom coefficients that was reached/1 -> Demux/1
  Demux/1 -> Moments/1(C_L)
  Demux/2 -> Moments/2(C_M)
  Demux/3 -> Moments/3(C_N)
  Bus Selector1/1 -> Moments/4(q)  "<q (Pa)>"
  Moments/1(L) -> Ang Accel/1(L)
  Moments/2(M) -> Ang Accel/2(M)
  Moments/3(N) -> Ang Accel/3(N)
  Bus Selector1/2 -> Ang Accel/4(omega_b)  "<omega_b meas (rad/s)>"
  Ang Accel/1(p_dot) -> Mux/1
  Ang Accel/3(r_dot) -> Mux/3
  Ang Accel/2(q_dot) -> Mux/2
  Bus Selector/6 -> Mux1/6  "<Throttle_meas>"
  Bus Selector/4 -> Mux1/4  "<SS meas (rad)>"
  Bus Selector/3 -> Mux1/3  "<AoA meas (rad)>"
  Bus Selector/2 -> Mux1/2  "<V_TAS (m/s)>"
  Bus Selector/1 -> Mux1/1  "<Alt meas (m)>"
  Bus Selector/5 -> Mux1/5  "<omega_b meas (rad/s)>"
  Mux1/1 -> Mom coefficients that was reached/1
  max deflections estimator/1(max_defl) -> Mux1/7

== system F16ASYM_Controlled/Primary Controller/P con + adaptive Crossed NN + AWU+Lim + Scheduling/Sigmoid  ==
  In : Inport
  Display : Display
  Fcn1 : Fcn  Commented=on  Expr=2.0 ./ (1.0 + exp(-u(4)*u(1:3)))-1
  MATLAB Function : MATLAB Function  TreatAsAtomicUnit=on
  a : Constant  Value=a
  Out : Outport
  wires:
  a/1 -> MATLAB Function/2(a)
  In/1 -> MATLAB Function/1(u)
  MATLAB Function/1(y) -> Out/1, Display/1

== system F16ASYM_Controlled/Primary Controller/P cont + adaptive Crossed NN + AWU+Lim /Body Rates Controller ==
  p_ref : Inport
  q_ref : Inport  Port=2
  r_ref : Inport  Port=3
  All_meas : Inport  Port=4
  Bus Creator : BusCreator
  Bus Creator1 : BusCreator
  Bus Creator2 : BusCreator
  Bus Selector : BusSelector  OutputSignals=signal1.omega_b meas (rad/s)
  Display1 : Display
  Mux : Mux  Inputs=3
  Ref Model and P Controller p : Adaptive_FaultTolerantControl/Ref Model and P Controller  tau=0.25  y_i=trim_state(10)  K_f=1  K_b=7
  Ref Model and P Controller q : Adaptive_FaultTolerantControl/Ref Model and P Controller  tau=0.06  y_i=trim_state(11)  K_f=1  K_b=3.5
  Ref Model and P Controller r : Adaptive_FaultTolerantControl/Ref Model and P Controller  tau=0.08  y_i=trim_state(12)  K_f=1  K_b=4
  Selector : Selector  InputPortWidth=3
  Selector1 : Selector  InputPortWidth=3  Indices=2
  Selector2 : Selector  InputPortWidth=3  Indices=3
  Sum : Sum  Inputs=+-|
  Sum1 : Sum  Inputs=+-|
  Sum2 : Sum  Inputs=+-|
  q_chanel vars : Outport
  p_chanel vars : Outport  Port=2
  r_chanel vars : Outport  Port=3
  Angular acc des (rad/s^2) : Outport  Port=4
  wires:
  All_meas/1 -> Bus Selector/1
  Bus Selector/1 -> Selector/1, Selector1/1, Selector2/1  "<omega_b meas (rad/s)>"
  p_ref/1 -> Ref Model and P Controller p/1
  Selector/1 -> Ref Model and P Controller p/2
  Ref Model and P Controller p/1 -> Mux/1
  Mux/1 -> Angular acc des (rad/s^2)/1
  q_ref/1 -> Ref Model and P Controller q/1
  Selector1/1 -> Ref Model and P Controller q/2
  r_ref/1 -> Ref Model and P Controller r/1
  Ref Model and P Controller q/1 -> Mux/2
  Ref Model and P Controller r/1 -> Mux/3
  Ref Model and P Controller p/2 -> Bus Creator/1  "p_sf_dot"
  Ref Model and P Controller p/3 -> Sum/1, Bus Creator/2  "p_sf"
  Sum/1 -> Display1/1, Bus Creator/3  "p_err"
  Bus Creator/1 -> p_chanel vars/1
  Bus Creator1/1 -> q_chanel vars/1
  Bus Creator2/1 -> r_chanel vars/1
  Selector2/1 -> Ref Model and P Controller r/2
  Ref Model and P Controller p/4 -> Sum/2
  Ref Model and P Controller p/5 -> Bus Creator/4  "K_b_p"
  Ref Model and P Controller q/2 -> Bus Creator1/1  "q_sf_dot"
  Ref Model and P Controller q/3 -> Sum1/1, Bus Creator1/2  "q_sf"
  Sum1/1 -> Bus Creator1/3  "q_err"
  Ref Model and P Controller q/4 -> Sum1/2
  Ref Model and P Controller q/5 -> Bus Creator1/4  "K_b_q"
  Ref Model and P Controller r/2 -> Bus Creator2/1  "r_sf_dot"
  Ref Model and P Controller r/3 -> Sum2/1, Bus Creator2/2  "r_sf"
  Sum2/1 -> Bus Creator2/3  "r_err"
  Ref Model and P Controller r/4 -> Sum2/2
  Ref Model and P Controller r/5 -> Bus Creator2/4  "K_b_r"

== system F16ASYM_Controlled/Primary Controller/P cont + adaptive Crossed NN + AWU+Lim /Complete crossed On-line (adaptive) multi-layer NN ==
  v_ad^ prev : Inport
  All_meas : Inport  Port=2
  NN variables : Inport  Port=3
  AWU : Inport  Port=4
  Complete crossed On-line (adaptive) multi-layer NN: A_w_z : Subsystem  VariantControl=NN on A_w_z
  Complete crossed On-line (adaptive) multi-layer NN: AoA : Subsystem  VariantControl=NN on AoA
  v_ad^ : Outport

== system F16ASYM_Controlled/Primary Controller/P cont + adaptive Crossed NN + AWU+Lim /Lat_dir Dyn Inversion: beta_dot->r_c ==
  beta_dot_c : Inport
  All_meas : Inport  Port=2
  A_w_y : Selector  InputPortWidth=3  Indices=2
  Bus Selector : BusSelector  OutputSignals=signal1.AoA meas (rad),signal1.omega_b meas (rad/s),signal1.V_TAS (m/s),signal2.A_w_CG
  Divide1 : Product  Inputs=**
  Divide3 : Product  Inputs=**
  Divide4 : Product  Inputs=/*
  Divide5 : Product  Inputs=*/
  Selector : Selector  InputPortWidth=3
  Trigonometric Function : Trigonometry  Operator=cos
  Trigonometric Function3 : Trigonometry  Operator=tan
  "q_c " : Sum  Inputs=-++
  r_c : Outport
  wires:
  "q_c "/1 -> r_c/1
  Bus Selector/1 -> Trigonometric Function/1, Trigonometric Function3/1  "<AoA meas (rad)>"
  Bus Selector/2 -> Selector/1  "<omega_b meas (rad/s)>"
  Divide1/1 -> "q_c "/2
  Divide3/1 -> Divide4/1
  A_w_y/1 -> Divide4/2
  All_meas/1 -> Bus Selector/1
  Bus Selector/4 -> A_w_y/1  "<A_w_CG>"
  Divide4/1 -> "q_c "/3
  Bus Selector/3 -> Divide3/2  "<V_TAS (m/s)>"
  Trigonometric Function/1 -> Divide3/1, Divide5/2
  Divide5/1 -> "q_c "/1
  beta_dot_c/1 -> Divide5/1
  Trigonometric Function3/1 -> Divide1/1
  Selector/1 -> Divide1/2

== system F16ASYM_Controlled/Primary Controller/P cont + adaptive Crossed NN + AWU+Lim /Long Dyn Inversion: alpha_dot ->q ==
  alpha_dot_c : Inport
  All_meas : Inport  Port=2
  Completed : Subsystem
  Manual Switch : ManualSwitch
  Simplified : Subsystem
  q_c : Outport
  wires:
  alpha_dot_c/1 -> Simplified/1(alpha_dot_c), Completed/1(alpha_dot_c)
  All_meas/1 -> Simplified/2(All_meas), Completed/2(All_meas)
  Completed/1(q_c) -> Manual Switch/1
  Simplified/1(q_c) -> Manual Switch/2
  Manual Switch/1 -> q_c/1

== system F16ASYM_Controlled/Primary Controller/P cont + adaptive Crossed NN + AWU+Lim /Longitudinal Controller: AoA or A_w_z ==
  A_w_z des : Inport
  AoA des (rad) : Inport  Port=2
  Anti-windup A_w_z : Inport  Port=3
  Anti-windup AoA : Inport  Port=4
  All meas : Inport  Port=5
  Longitudinal controller in A_w_z : Subsystem  VariantControl=Controller of A_w_z
  Longitudinal controller in AoA : Subsystem  VariantControl=Controller of AoA
  A_chanel vars : Outport
  alpha_chanel vars : Outport  Port=2
  alpha_dot_c : Outport  Port=3

== system F16ASYM_Controlled/Primary Controller/P cont + adaptive Crossed NN + AWU+Lim /Physical limitation ==
  note: Converto to Angular accelerations
  v comm : Inport
  all meas : Inport  Port=2
  Ang Accel : MATLAB Function
  Bus Selector : BusSelector  OutputSignals=signal1.Alt meas (m),signal1.V_TAS (m/s),signal1.AoA meas (rad),signal1.SS meas (rad),signal1.omega_b meas (rad/s),signal1.Throttle_meas
  Bus Selector1 : BusSelector  OutputSignals=signal2.q (Pa),signal1.omega_b meas (rad/s)
  Demux : Demux  Outputs=3
  Display : Display
  Display1 : Display
  Display2 : Display
  Divide : Product  Inputs=**
  Divide1 : Product  Inputs=**
  Gain : Gain  Gain=-1
  Gain1 : Gain
  Mom coefficients that can be reached : MATLABFcn  MATLABFcn=Moms_Coeff_estimator  OutputDimensions=3  OutputSignalType=real
  Moments : Subsystem
  Mux : Mux  Inputs=3
  Mux1 : Mux  Inputs=7
  Saturation Dynamic : simulink/Discontinuities/Saturation Dynamic  OutMin=[]  OutMax=[]  OutDataTypeStr=Inherit: Same as second input  OutDataType=fixdt(1, 16)  OutScaling=2^-10  DoSatur=off
  Sign : Signum
  Sign1 : Signum
  max deflections estimator : MATLAB Function  TreatAsAtomicUnit=on
  v limted : Outport
  wires:
  max deflections estimator/1(max_defl) -> Mux1/7
  Mux1/1 -> Mom coefficients that can be reached/1
  Bus Selector/5 -> Mux1/5  "<omega_b meas (rad/s)>"
  Bus Selector/1 -> Mux1/1  "<Alt meas (m)>"
  Bus Selector/2 -> Mux1/2  "<V_TAS (m/s)>"
  Bus Selector/3 -> Mux1/3  "<AoA meas (rad)>"
  Bus Selector/4 -> Mux1/4  "<SS meas (rad)>"
  Bus Selector/6 -> Mux1/6  "<Throttle_meas>"
  Ang Accel/2(q_dot) -> Mux/2
  Ang Accel/3(r_dot) -> Mux/3
  Ang Accel/1(p_dot) -> Mux/1
  Bus Selector1/2 -> Ang Accel/4(omega_b)  "<omega_b meas (rad/s)>"
  Moments/3(N) -> Ang Accel/3(N)
  Moments/2(M) -> Ang Accel/2(M)
  Moments/1(L) -> Ang Accel/1(L)
  Bus Selector1/1 -> Moments/4(q)  "<q (Pa)>"
  Demux/3 -> Moments/3(C_N)
  Demux/2 -> Moments/2(C_M)
  Demux/1 -> Moments/1(C_L)
  Mom coefficients that can be reached/1 -> Demux/1
  all meas/1 -> Bus Selector/1, Bus Selector1/1
  Mux/1 -> Gain1/1
  v comm/1 -> Saturation Dynamic/2, Display1/1, max deflections estimator/1(v_comm)
  Saturation Dynamic/1 -> Display/1, v limted/1
  Sign/1 -> Divide/1
  Gain1/1 -> Divide/2, Divide1/1, Sign1/1, Display2/1, Sign/1
  Sign1/1 -> Gain/1
  Divide/1 -> Saturation Dynamic/1
  Gain/1 -> Divide1/2
  Divide1/1 -> Saturation Dynamic/3

== system F16ASYM_Controlled/Primary Controller/P cont + adaptive Crossed NN + AWU+Lim /Sigmoid  ==
  In : Inport
  Display : Display
  Fcn1 : Fcn  Commented=on  Expr=2.0 ./ (1.0 + exp(-u(4)*u(1:3)))-1
  MATLAB Function : MATLAB Function  TreatAsAtomicUnit=on
  a : Constant  Value=a
  Out : Outport
  wires:
  MATLAB Function/1(y) -> Display/1, Out/1
  In/1 -> MATLAB Function/1(u)
  a/1 -> MATLAB Function/2(a)

== system F16ASYM_Controlled/Primary Controller/P cont + adaptive Crossed NN + AWU+Lim ONELAYER/Body Rates Controller ==
  p_ref : Inport
  q_ref : Inport  Port=2
  r_ref : Inport  Port=3
  All_meas : Inport  Port=4
  Bus Creator : BusCreator
  Bus Creator1 : BusCreator
  Bus Creator2 : BusCreator
  Bus Selector : BusSelector  OutputSignals=signal1.omega_b meas (rad/s)
  Display1 : Display
  Mux : Mux  Inputs=3
  Ref Model and P Controller p : Adaptive_FaultTolerantControl/Ref Model and P Controller  tau=0.25  y_i=trim_state(10)  K_f=1  K_b=7
  Ref Model and P Controller q : Adaptive_FaultTolerantControl/Ref Model and P Controller  tau=0.06  y_i=trim_state(11)  K_f=1  K_b=3.5
  Ref Model and P Controller r : Adaptive_FaultTolerantControl/Ref Model and P Controller  tau=0.08  y_i=trim_state(12)  K_f=1  K_b=4
  Selector : Selector  InputPortWidth=3
  Selector1 : Selector  InputPortWidth=3  Indices=2
  Selector2 : Selector  InputPortWidth=3  Indices=3
  Sum : Sum  Inputs=+-|
  Sum1 : Sum  Inputs=+-|
  Sum2 : Sum  Inputs=+-|
  q_chanel vars : Outport
  p_chanel vars : Outport  Port=2
  r_chanel vars : Outport  Port=3
  Angular acc des (rad/s^2) : Outport  Port=4
  wires:
  All_meas/1 -> Bus Selector/1
  Bus Selector/1 -> Selector/1, Selector1/1, Selector2/1  "<omega_b meas (rad/s)>"
  p_ref/1 -> Ref Model and P Controller p/1
  Selector/1 -> Ref Model and P Controller p/2
  Ref Model and P Controller p/1 -> Mux/1
  Mux/1 -> Angular acc des (rad/s^2)/1
  q_ref/1 -> Ref Model and P Controller q/1
  Selector1/1 -> Ref Model and P Controller q/2
  r_ref/1 -> Ref Model and P Controller r/1
  Ref Model and P Controller q/1 -> Mux/2
  Ref Model and P Controller r/1 -> Mux/3
  Ref Model and P Controller p/2 -> Bus Creator/1  "p_sf_dot"
  Ref Model and P Controller p/3 -> Sum/1, Bus Creator/2  "p_sf"
  Sum/1 -> Display1/1, Bus Creator/3  "p_err"
  Bus Creator/1 -> p_chanel vars/1
  Bus Creator1/1 -> q_chanel vars/1
  Bus Creator2/1 -> r_chanel vars/1
  Selector2/1 -> Ref Model and P Controller r/2
  Ref Model and P Controller p/4 -> Sum/2
  Ref Model and P Controller p/5 -> Bus Creator/4  "K_b_p"
  Ref Model and P Controller q/2 -> Bus Creator1/1  "q_sf_dot"
  Ref Model and P Controller q/3 -> Sum1/1, Bus Creator1/2  "q_sf"
  Sum1/1 -> Bus Creator1/3  "q_err"
  Ref Model and P Controller q/4 -> Sum1/2
  Ref Model and P Controller q/5 -> Bus Creator1/4  "K_b_q"
  Ref Model and P Controller r/2 -> Bus Creator2/1  "r_sf_dot"
  Ref Model and P Controller r/3 -> Sum2/1, Bus Creator2/2  "r_sf"
  Sum2/1 -> Bus Creator2/3  "r_err"
  Ref Model and P Controller r/4 -> Sum2/2
  Ref Model and P Controller r/5 -> Bus Creator2/4  "K_b_r"

== system F16ASYM_Controlled/Primary Controller/P cont + adaptive Crossed NN + AWU+Lim ONELAYER/Complete crossed On-line (adaptive) multi-layer NN ==
  v_ad^ prev : Inport
  All_meas : Inport  Port=2
  NN variables : Inport  Port=3
  AWU : Inport  Port=4
  Complete crossed On-line (adaptive) multi-layer NN: A_w_z : Subsystem  VariantControl=NN on A_w_z
  Complete crossed On-line (adaptive) multi-layer NN: AoA : Subsystem  VariantControl=NN on AoA
  v_ad^ : Outport

== system F16ASYM_Controlled/Primary Controller/P cont + adaptive Crossed NN + AWU+Lim ONELAYER/Lat_dir Dyn Inversion: beta_dot->r_c ==
  beta_dot_c : Inport
  All_meas : Inport  Port=2
  A_w_y : Selector  InputPortWidth=3  Indices=2
  Bus Selector : BusSelector  OutputSignals=signal1.AoA meas (rad),signal1.omega_b meas (rad/s),signal1.V_TAS (m/s),signal2.A_w_CG
  Divide1 : Product  Inputs=**
  Divide3 : Product  Inputs=**
  Divide4 : Product  Inputs=/*
  Divide5 : Product  Inputs=*/
  Selector : Selector  InputPortWidth=3
  Trigonometric Function : Trigonometry  Operator=cos
  Trigonometric Function3 : Trigonometry  Operator=tan
  "q_c " : Sum  Inputs=-++
  r_c : Outport
  wires:
  "q_c "/1 -> r_c/1
  Bus Selector/1 -> Trigonometric Function/1, Trigonometric Function3/1  "<AoA meas (rad)>"
  Bus Selector/2 -> Selector/1  "<omega_b meas (rad/s)>"
  Divide1/1 -> "q_c "/2
  Divide3/1 -> Divide4/1
  A_w_y/1 -> Divide4/2
  All_meas/1 -> Bus Selector/1
  Bus Selector/4 -> A_w_y/1  "<A_w_CG>"
  Divide4/1 -> "q_c "/3
  Bus Selector/3 -> Divide3/2  "<V_TAS (m/s)>"
  Trigonometric Function/1 -> Divide3/1, Divide5/2
  Divide5/1 -> "q_c "/1
  beta_dot_c/1 -> Divide5/1
  Trigonometric Function3/1 -> Divide1/1
  Selector/1 -> Divide1/2

== system F16ASYM_Controlled/Primary Controller/P cont + adaptive Crossed NN + AWU+Lim ONELAYER/Long Dyn Inversion: alpha_dot ->q ==
  alpha_dot_c : Inport
  All_meas : Inport  Port=2
  Completed : Subsystem
  Manual Switch : ManualSwitch
  Simplified : Subsystem
  q_c : Outport
  wires:
  alpha_dot_c/1 -> Simplified/1(alpha_dot_c), Completed/1(alpha_dot_c)
  All_meas/1 -> Simplified/2(All_meas), Completed/2(All_meas)
  Completed/1(q_c) -> Manual Switch/1
  Simplified/1(q_c) -> Manual Switch/2
  Manual Switch/1 -> q_c/1

== system F16ASYM_Controlled/Primary Controller/P cont + adaptive Crossed NN + AWU+Lim ONELAYER/Longitudinal Controller: AoA or A_w_z ==
  A_w_z des : Inport
  AoA des (rad) : Inport  Port=2
  Anti-windup A_w_z : Inport  Port=3
  Anti-windup AoA : Inport  Port=4
  All meas : Inport  Port=5
  Longitudinal controller in A_w_z : Subsystem  VariantControl=Controller of A_w_z
  Longitudinal controller in AoA : Subsystem  VariantControl=Controller of AoA
  A_chanel vars : Outport
  alpha_chanel vars : Outport  Port=2
  alpha_dot_c : Outport  Port=3
